simulink model "Identified_model"  (R2023b)
settings: Solver=VariableStepAuto  StartTime=0.0  StopTime=10.0  RelTol=1e-3
values from neighbouring files (symbols this model uses):
  b = 2.1E-5    (= 2.1e-05)    [motor_constants.m]
  bg = 1E-5    (= 1e-05)    [motor_constants.m]
  J = 1.8E-5    (= 1.8e-05)    [motor_constants.m]
  ke = 0.05    [motor_constants.m]
  keg = 0.09    [motor_constants.m]
  km = 0.18    [motor_constants.m]
  kmg = 0.12    [motor_constants.m]
  L = 0.3    [motor_constants.m]
  Lg = 0.1    [motor_constants.m]
  R = 5    [motor_constants.m]
  Rg = 1    [motor_constants.m]
  u_max = 10    [motor_constants.m]
  u_min = -u_max    (= -10)    [motor_constants.m]
  un = 0.8    [motor_constants.m]
settings Model: Creator=Lenovo  LastModifiedBy=Lenovo

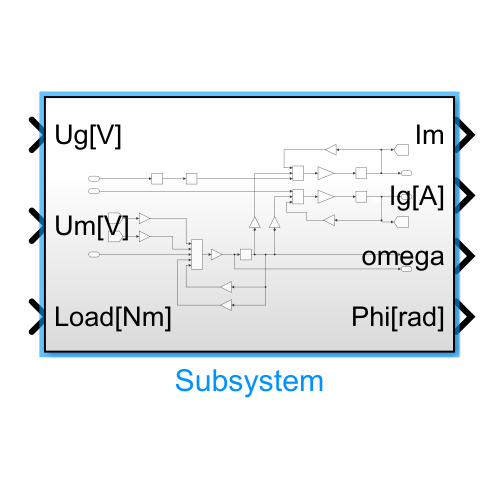
[thumbnail: Simulink's stored preview of the top-level diagram]
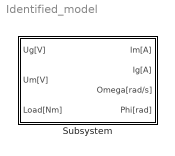
== system Identified_model ==
  Subsystem : Subsystem

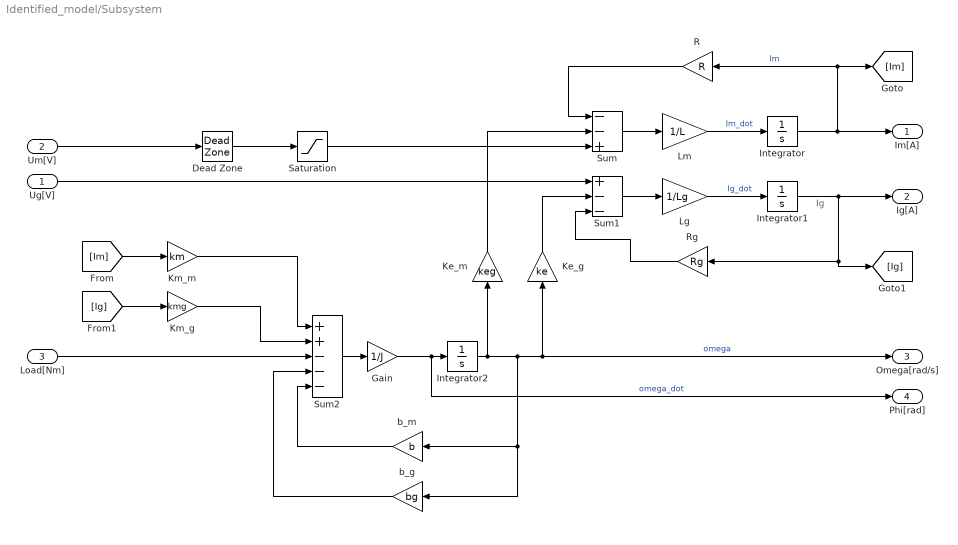
== system Identified_model/Subsystem ==
  note: Ig
  Ug[V] : Inport
  Um[V] : Inport  Port=2
  Load[Nm] : Inport  Port=3
  Dead Zone : DeadZone  LowerValue=-un  UpperValue=un
  Gain : Gain  Gain=1/J
  Integrator : Integrator
  Integrator1 : Integrator
  Integrator2 : Integrator
  Ke_g : Gain  Gain=ke
  Ke_m : Gain  Gain=keg
  Km_g : Gain  Gain=kmg
  Km_m : Gain  Gain=km
  Lg : Gain  Gain=1/Lg
  Lm : Gain  Gain=1/L
  R : Gain  Gain=R
  Rg : Gain  Gain=Rg
  Saturation : Saturate  UpperLimit=u_max  LowerLimit=u_min
  Sum : Sum  Inputs=--+
  Sum1 : Sum  Inputs=+--
  Sum2 : Sum  Inputs=++---
  b_g : Gain  Gain=bg
  b_m : Gain  Gain=b
  Im[A] : Outport
  Ig[A] : Outport  Port=2
  Omega[rad/s] : Outport  Port=3
  Phi[rad] : Outport  Port=4
  wires:
  Integrator/1 -> Im[A]/1, [Im], R/1  "Im"
  Um[V]/1 -> Dead Zone/1
  [Im] -> Km_m/1
  Lm/1 -> Integrator/1  "Im_dot"
  Integrator2/1 -> Omega[rad/s]/1, Ke_g/1, b_g/1, b_m/1, Ke_m/1  "omega"
  [Ig] -> Km_g/1
  Km_m/1 -> Sum2/1
  Integrator1/1 -> Ig[A]/1, [Ig], Rg/1
  Sum2/1 -> Gain/1
  Sum/1 -> Lm/1
  Km_g/1 -> Sum2/2
  Rg/1 -> Sum1/3
  R/1 -> Sum/1
  Ug[V]/1 -> Sum1/1
  Ke_m/1 -> Sum/2
  b_m/1 -> Sum2/5
  Ke_g/1 -> Sum1/2
  Lg/1 -> Integrator1/1  "Ig_dot"
  Sum1/1 -> Lg/1
  b_g/1 -> Sum2/4
  Load[Nm]/1 -> Sum2/3
  Gain/1 -> Phi[rad]/1, Integrator2/1  "omega_dot"
  Dead Zone/1 -> Saturation/1
  Saturation/1 -> Sum/3
